simulink model "dtmf"  (Simulink 6.1)
settings: Solver=VariableStepDiscrete  StartTime=0  StopTime=5  RelTol=1e-3
PreLoadFcn:
  | Framesize=256,Fs=8192
values from neighbouring files (symbols this model uses):
  Fs = 8000    [generate.m]
undefined symbols (not defined in the file or in its folder): jet
libraries: dspddes3 x14, dspsrcs3 x5, dspsrcs2 x3, simulink3 x3, commutil2 x2, dspsigattribs x2, dspsigops x1, dsparch3 x1, dspswit3 x1, dspbuff3 x1, dspspect3 x1, dspsnks3 x1
settings Model: Creator=stuartm  LastModifiedBy=y  ExtModeTrigMode=oneshot  ExtModeArmWhenConnect=off  BufferReuse=off
settings DataIOCC: LimitDataPoints=off
settings OptimizationCC: BlockReduction=off  BooleanDataType=off  InlineInvariantSignals=off  OptimizeBlockIOStorage=off  BufferReuse=off  EnforceIntegerDowncast=off  ExpressionFolding=off  FoldNonRolledExpr=off  LocalBlockOutputs=off
settings HardwareCC: TargetUnknown=on

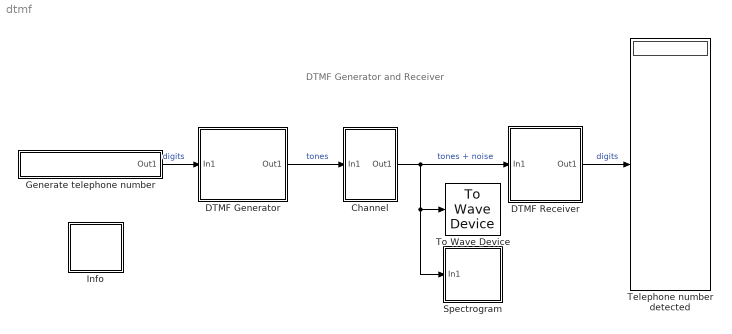
== system dtmf ==
  note: DTMF Generator and Receiver
  Channel : Subsystem  mask{var=.04, Fs=Fs, Framesize=Framesize, g=2}
      mask prompts: var "Noise power"; Fs "Sample Rate (Hz)"; g "Gain"
      mask Display: disp('Channel')
  DTMF Generator : Subsystem  mask{Fs=Fs, Framesize=Framesize}
      mask prompts: Fs "Sample Rate (Hz)"; Framesize "Framesize (Samples)"
      mask Display: disp('DTMF\nGenerator')
  DTMF Receiver : Subsystem  mask{Fs=Fs, Framesize=Framesize}
      mask prompts: Fs "Sample Rate"
      mask Display: disp('DTMF\nReceiver');
  Generate telephone number : Subsystem  mask{Number=[1 8 0 0 6 5 3 1 4 1 5], Td=(1/Fs)*256*6}
      mask prompts: Number "Telephone number"; Td "Digit Period (s)"
      mask Display: disp(Number)
  Info : Subsystem
      mask Display: disp('Info');
  Spectrogram : Subsystem
  Telephone number detected : Display
  To Wave Device : dspwin32/To Wave Device  bufDuration=1  initDelay=0.3  useDefaultDevice=on  userDeviceID=SoundMAX Digital Audio  enable24Bit=off
  wires:
  DTMF Generator/1(Out1) -> Channel/1(In1)  "tones"
  Generate telephone number/1(Out1) -> DTMF Generator/1(In1)  "digits"
  Channel/1(Out1) -> DTMF Receiver/1(In1), To Wave Device/1, Spectrogram/1(In1)  "tones + noise"
  DTMF Receiver/1(Out1) -> Telephone number detected/1  "digits"

== system dtmf/Channel ==
  In1 : Inport  Port=1  LatchInput=off
  Gain : Gain  Gain=g  SaturateOnIntegerOverflow=on
  Sum : Sum  Inputs=|++  SaturateOnIntegerOverflow=on  InputSameDT=on
  Vector of Noise : RandomNumber  Variance=var  Seed=[1:Framesize]  SampleTime=Framesize/Fs
  Out1 : Outport
  wires:
  In1/1 -> Gain/1
  Gain/1 -> Sum/1
  Vector of Noise/1 -> Sum/2
  Sum/1 -> Out1/1

== system dtmf/DTMF Generator ==
  In1 : Inport  Port=1  LatchInput=off
  Digit to Tone : Subsystem  TreatAsAtomicUnit=on
  Subtract  1 : Subsystem
  Out1 : Outport
  wires:
  Subtract  1/1(Out1) -> Digit to Tone/1(In1)
  In1/1 -> Subtract  1/1(In1), Digit to Tone/Enable
  Digit to Tone/1(Out1) -> Out1/1

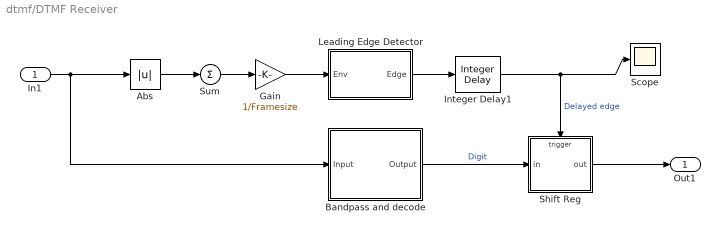
== system dtmf/DTMF Receiver ==
  In1 : Inport  Port=1  LatchInput=off
  Abs : Abs  SaturateOnIntegerOverflow=on
  Bandpass and decode : Subsystem
  Gain : Gain  Gain=1/Framesize  SaturateOnIntegerOverflow=on
  Integer Delay1 : dspsigops/Integer Delay  delay=1  ic=0
  Leading Edge Detector : Subsystem
  Scope : Scope
  Shift Reg : Stateflow chart  TreatAsAtomicUnit=on
  Sum : Sum  Inputs=1  SaturateOnIntegerOverflow=on  InputSameDT=on
  Out1 : Outport
  wires:
  In1/1 -> Bandpass and decode/1(Input), Abs/1
  Abs/1 -> Sum/1
  Sum/1 -> Gain/1
  Gain/1 -> Leading Edge Detector/1(Env)
  Shift Reg/1(out) -> Out1/1
  Integer Delay1/1 -> Shift Reg/Trigger, Scope/1  "Delayed edge"
  Bandpass and decode/1(Output) -> Shift Reg/1(in)  "Digit"
  Leading Edge Detector/1(Edge) -> Integer Delay1/1

== system dtmf/Generate telephone number ==
  Discrete Pulse Generator : DiscretePulseGenerator  SampleTime=Td
  Product : Product  SaturateOnIntegerOverflow=on  RndMeth=Zero  InputSameDT=on
  Triggered Signal From Workspace1 : dspsrcs3/Triggered Signal From Workspace  Signal=Number+1  TriggerType=Rising edge  ic=0  SamplesPerFrame=1  OutputAfterFinalValue=Setting To Zero
  Out1 : Outport
  wires:
  Discrete Pulse Generator/1 -> Product/1, Triggered Signal From Workspace1/Trigger
  Triggered Signal From Workspace1/1 -> Product/2
  Product/1 -> Out1/1

== system dtmf/Info ==
  note: DTMF Generator and Receiver
  note: This system uses the bandpass filter method of DTMF reception
      |
      | Enter a telephone number in first block
      |
      | "Telephone number detected" block shows last 12 digits detected

== system dtmf/Spectrogram ==
  In1 : Inport  Port=1  LatchInput=off
  Buffer2 : dspbuff3/Buffer  N=48  V=46  ic=-70
  Selector : Selector  Elements=1:Framesize/4  InputPortWidth=Framesize/2
  Short-Time FFT1 : dspspect3/Short-Time FFT  wintype=Hamming  Rs=50  beta=5  winsamp=Periodic  inheritFFT=off  fftsize=128  navg=2
  Spectogram : dspsnks3/Matrix Viewer  ImageParams=on  CMapStr=jet(256)  AxisColorbar=off  AxisParams=on  AxisOrigin=Lower left corner  XLabel=Time Index  YLabel=Frequency Index  ZLabel=dB Magnitude  FigPos=[54 474 312 203]  AxisZoom=off
      settings: YMin=-81.1042710009338  YMax=33.5779095386242
  To Workspace : ToWorkspace  VariableName=tones  SampleTime=-1  SaveFormat=Array
  Transpose : dspmtrx3/Transpose  Hermitian=off
  dB Conversion : dspmathops/dB Conversion  dBtype=dB  intype=Amplitude  R=1  fuzz=on
  wires:
  Short-Time FFT1/1 -> Selector/1
  Selector/1 -> dB Conversion/1
  Buffer2/1 -> Transpose/1
  dB Conversion/1 -> Buffer2/1
  In1/1 -> Short-Time FFT1/1, To Workspace/1
  Transpose/1 -> Spectogram/1

== system dtmf/DTMF Generator/Digit to Tone ==
  In1 : Inport  Port=1  LatchInput=off
  Enable : EnablePort
  Column Tones 1209Hz 1336Hz 1477Hz : Subsystem
  Column value for digit : Lookup  DialogController=Simulink.DDGSource  InputValues=[0 1 2 3 4 5 6 7 8 9 10 11]  OutputValues=[1 0 1 2 0 1 2 0 1 2 0 2]  SaturateOnIntegerOverflow=on
  "Row Tones 697Hz 770Hz 852Hz 941Hz " : Subsystem
  Row value for digit : Lookup  DialogController=Simulink.DDGSource  InputValues=[0 1 2 3 4 5 6 7 8 9 10 11]  OutputValues=[3 0 0 0 1 1 1 2 2 2 3 3]  SaturateOnIntegerOverflow=on
  Sum : Sum  Inputs=|+-  SaturateOnIntegerOverflow=on  InputSameDT=on
  Out1 : Outport  OutputWhenDisabled=reset  InitialOutput=0
  wires:
  Sum/1 -> Out1/1
  Column value for digit/1 -> Column Tones 1209Hz 1336Hz 1477Hz/1(Column)
  Row value for digit/1 -> "Row Tones 697Hz 770Hz 852Hz 941Hz "/1(Row)
  In1/1 -> Column value for digit/1, Row value for digit/1
  Column Tones 1209Hz 1336Hz 1477Hz/1(Tone) -> Sum/2
  "Row Tones 697Hz 770Hz 852Hz 941Hz "/1(Tone) -> Sum/1

== system dtmf/DTMF Generator/Subtract  1 ==
  In1 : Inport  Port=1  LatchInput=off
  Constant : Constant
  Sum : Sum  Inputs=|+-  SaturateOnIntegerOverflow=on  InputSameDT=on
  Out1 : Outport
  wires:
  Sum/1 -> Out1/1
  In1/1 -> Sum/1
  Constant/1 -> Sum/2

== system dtmf/DTMF Receiver/Bandpass and decode ==
  Input : Inport  Port=1  LatchInput=off
  Calculate Digit : simulink3/Functions & Tables/Look-Up Table (2-D)  x=[1:4]  y=[1:3]  t=[1 2 3;4 5 6;7 8 9;10 0 11]
  Calculate Column : Subsystem
  Calculate Row : Subsystem
  Output : Outport
  wires:
  Input/1 -> Calculate Column/1(In1), Calculate Row/1(In1)  "Input Tones"
  Calculate Digit/1 -> Output/1
  Calculate Row/1(Out1) -> Calculate Digit/1
  Calculate Column/1(Out1) -> Calculate Digit/2

== system dtmf/DTMF Receiver/Leading Edge Detector ==
  Env : Inport  Port=1  LatchInput=off
  Binary To Bipolar : Fcn  Expr=2*u-1
  Constant : Constant  Value=0.5
  Direct-Form II Transpose Filter : dsparch3/Direct-Form II Transpose Filter  num=[ones(1,4) -ones(1,4)]  den=1  ic=0
  Edge Detector1 : dspswit3/Edge Detector
  Relational Operator : RelationalOperator  InputSameDT=on
  Rising Edge Start : Fcn  Expr=u>5
  Edge : Outport  InitialOutput=0
  wires:
  Edge Detector1/1 -> Edge/1
  Direct-Form II Transpose Filter/1 -> Rising Edge Start/1
  Binary To Bipolar/1 -> Direct-Form II Transpose Filter/1
  Rising Edge Start/1 -> Edge Detector1/1
  Env/1 -> Relational Operator/1
  Constant/1 -> Relational Operator/2
  Relational Operator/1 -> Binary To Bipolar/1

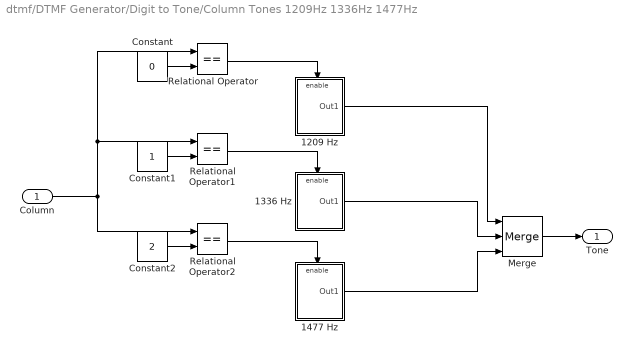
== system dtmf/DTMF Generator/Digit to Tone/Column Tones 1209Hz 1336Hz 1477Hz ==
  Column : Inport  Port=1  LatchInput=off
  1209 Hz : Subsystem  TreatAsAtomicUnit=on
  1336 Hz : Subsystem  TreatAsAtomicUnit=on
  1477 Hz : Subsystem  TreatAsAtomicUnit=on
  Constant : Constant  Value=0
  Constant1 : Constant
  Constant2 : Constant  Value=2
  Merge : Merge  Inputs=3
  Relational Operator : RelationalOperator  Operator===  InputSameDT=on
  Relational Operator1 : RelationalOperator  Operator===  InputSameDT=on
  Relational Operator2 : RelationalOperator  Operator===  InputSameDT=on
  Tone : Outport
  wires:
  Merge/1 -> Tone/1
  1477 Hz/1(Out1) -> Merge/3
  1336 Hz/1(Out1) -> Merge/2
  1209 Hz/1(Out1) -> Merge/1
  Column/1 -> Relational Operator/1, Relational Operator1/1, Relational Operator2/1
  Relational Operator/1 -> 1209 Hz/Enable
  Relational Operator1/1 -> 1336 Hz/Enable
  Relational Operator2/1 -> 1477 Hz/Enable
  Constant/1 -> Relational Operator/2
  Constant1/1 -> Relational Operator1/2
  Constant2/1 -> Relational Operator2/2

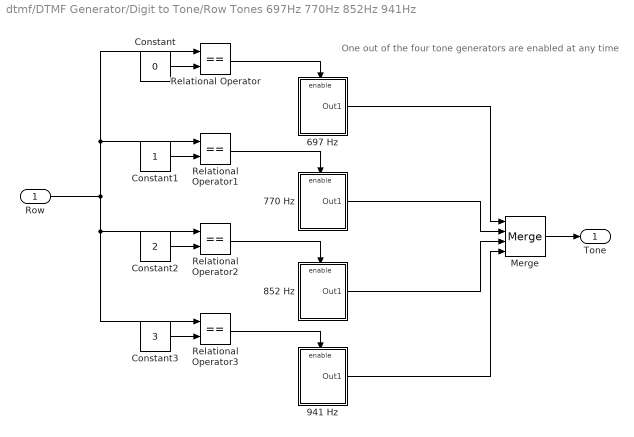
== system dtmf/DTMF Generator/Digit to Tone/Row Tones 697Hz 770Hz 852Hz 941Hz  ==
  note: One out of the four tone generators
      | are enabled at any time
  Row : Inport  Port=1  LatchInput=off
  697 Hz : Subsystem  TreatAsAtomicUnit=on
  770 Hz : Subsystem  TreatAsAtomicUnit=on
  852 Hz : Subsystem  TreatAsAtomicUnit=on
  941 Hz : Subsystem  TreatAsAtomicUnit=on
  Constant : Constant  Value=0
  Constant1 : Constant
  Constant2 : Constant  Value=2
  Constant3 : Constant  Value=3
  Merge : Merge  Inputs=4
  Relational Operator{,1..3} (4 alike) : RelationalOperator  Operator===  InputSameDT=on
  Tone : Outport
  wires:
  Row/1 -> Relational Operator/1, Relational Operator1/1, Relational Operator2/1, Relational Operator3/1
  697 Hz/1(Out1) -> Merge/1
  770 Hz/1(Out1) -> Merge/2
  852 Hz/1(Out1) -> Merge/3
  941 Hz/1(Out1) -> Merge/4
  Merge/1 -> Tone/1
  Relational Operator/1 -> 697 Hz/Enable
  Relational Operator1/1 -> 770 Hz/Enable
  Relational Operator2/1 -> 852 Hz/Enable
  Relational Operator3/1 -> 941 Hz/Enable
  Constant/1 -> Relational Operator/2
  Constant1/1 -> Relational Operator1/2
  Constant2/1 -> Relational Operator2/2
  Constant3/1 -> Relational Operator3/2

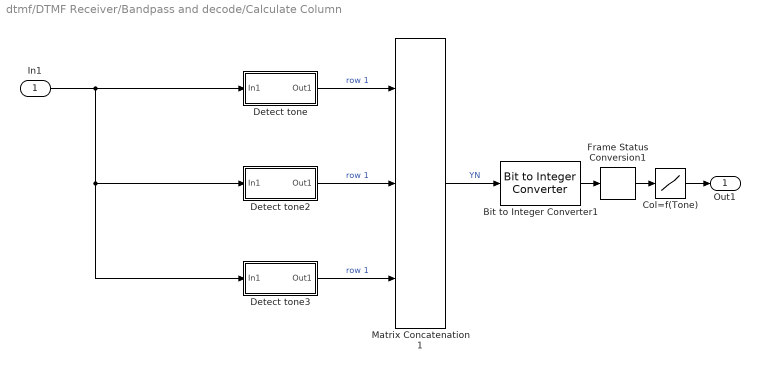
== system dtmf/DTMF Receiver/Bandpass and decode/Calculate Column ==
  In1 : Inport  Port=1  LatchInput=off
  Bit to Integer Converter1 : commutil2/Bit to Integer Converter  nbits=3
  Col=f(Tone) : Lookup  DialogController=Simulink.DDGSource  InputValues=[0:7]  OutputValues=[0 1 2 0 3 0 0 0]  SaturateOnIntegerOverflow=on
  Detect tone : Subsystem  mask{Fs=Fs, F=1477}
      mask prompts: Fs "Sample Rate (Hz)"; F "Frequency"
      settings: AttributesFormatString=%<F> Hz
  Detect tone2 : Subsystem  mask{Fs=Fs, F=1336}
      mask prompts: Fs "Sample Rate (Hz)"; F "Frequency"
      settings: AttributesFormatString=%<F> Hz
  Detect tone3 : Subsystem  mask{Fs=Fs, F=1209}
      mask prompts: Fs "Sample Rate (Hz)"; F "Frequency"
      settings: AttributesFormatString=%<F> Hz
  Frame Status Conversion1 : dspsigattribs/Frame Status Conversion  growRefPort=off  outframe=Sample-based
  Matrix Concatenation1 : simulink3/Signals & Systems/Matrix Concatenation  numInports=3  catMethod=Vertical
  Out1 : Outport
  wires:
  Matrix Concatenation1/1 -> Bit to Integer Converter1/1  "YN"
  Bit to Integer Converter1/1 -> Frame Status Conversion1/1
  Frame Status Conversion1/1 -> Col=f(Tone)/1
  Detect tone/1(Out1) -> Matrix Concatenation1/1  "row 1"
  Detect tone2/1(Out1) -> Matrix Concatenation1/2  "row 1"
  Detect tone3/1(Out1) -> Matrix Concatenation1/3  "row 1"
  In1/1 -> Detect tone2/1(In1), Detect tone3/1(In1), Detect tone/1(In1)
  Col=f(Tone)/1 -> Out1/1

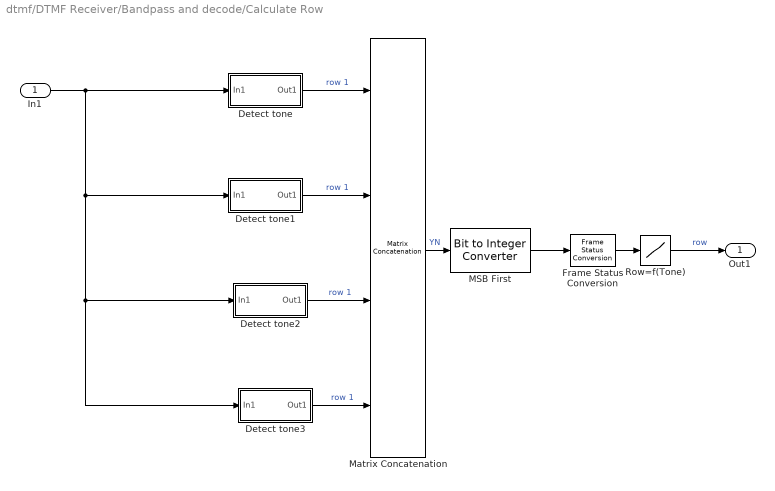
== system dtmf/DTMF Receiver/Bandpass and decode/Calculate Row ==
  In1 : Inport  Port=1  LatchInput=off
  Detect tone : Subsystem  mask{Fs=Fs, F=941}
      mask prompts: Fs "Sample Rate (Hz)"; F "Frequency"
      settings: AttributesFormatString=%<F> Hz
  Detect tone1 : Subsystem  mask{Fs=Fs, F=852}
      mask prompts: Fs "Sample Rate (Hz)"; F "Frequency"
      settings: AttributesFormatString=%<F> Hz
  Detect tone2 : Subsystem  mask{Fs=Fs, F=770}
      mask prompts: Fs "Sample Rate (Hz)"; F "Frequency"
      settings: AttributesFormatString=%<F> Hz
  Detect tone3 : Subsystem  mask{Fs=Fs, F=697}
      mask prompts: Fs "Sample Rate (Hz)"; F "Frequency"
      settings: AttributesFormatString=%<F> Hz
  Frame Status Conversion : dspsigattribs/Frame Status Conversion  growRefPort=off  outframe=Sample-based
  MSB First : commutil2/Bit to Integer Converter  nbits=4
  Matrix Concatenation : simulink3/Signals & Systems/Matrix Concatenation  numInports=4  catMethod=Vertical
  Row=f(Tone) : Lookup  DialogController=Simulink.DDGSource  InputValues=[0:15]  OutputValues=[0 1 2 0 3 0 0 0 4 0 0 0 0 0 0 0]  SaturateOnIntegerOverflow=on
  Out1 : Outport
  wires:
  Detect tone/1(Out1) -> Matrix Concatenation/1  "row 1"
  Matrix Concatenation/1 -> MSB First/1  "YN"
  MSB First/1 -> Frame Status Conversion/1
  Frame Status Conversion/1 -> Row=f(Tone)/1
  Detect tone1/1(Out1) -> Matrix Concatenation/2  "row 1"
  Detect tone2/1(Out1) -> Matrix Concatenation/3  "row 1"
  Detect tone3/1(Out1) -> Matrix Concatenation/4  "row 1"
  In1/1 -> Detect tone/1(In1), Detect tone1/1(In1), Detect tone2/1(In1), Detect tone3/1(In1)
  Row=f(Tone)/1 -> Out1/1  "row"

== system dtmf/DTMF Generator/Digit to Tone/Column Tones 1209Hz 1336Hz 1477Hz/1209 Hz ==
  Enable : EnablePort
  Sine Wave : dspsrcs2/Sine Wave  Amplitude=1  Frequency=1209  Phase=0  SampleMode=Discrete  OutComplex=Real  CompMethod=Trigonometric Fcn  SampleTime=1/Fs  SamplesPerFrame=Framesize  ResetState=Restart at time zero
  Out1 : Outport
  wires:
  Sine Wave/1 -> Out1/1

== system dtmf/DTMF Generator/Digit to Tone/Column Tones 1209Hz 1336Hz 1477Hz/1336 Hz ==
  Enable : EnablePort
  1336 Hz1 : dspsrcs2/Sine Wave  Amplitude=1  Frequency=1336  Phase=0  SampleMode=Discrete  OutComplex=Real  CompMethod=Trigonometric Fcn  SampleTime=1/Fs  SamplesPerFrame=Framesize  ResetState=Restart at time zero
  Out1 : Outport
  wires:
  1336 Hz1/1 -> Out1/1

== system dtmf/DTMF Generator/Digit to Tone/Column Tones 1209Hz 1336Hz 1477Hz/1477 Hz ==
  Enable : EnablePort
  1477 Hz1 : dspsrcs2/Sine Wave  Amplitude=1  Frequency=1477  Phase=0  SampleMode=Discrete  OutComplex=Real  CompMethod=Trigonometric Fcn  SampleTime=1/Fs  SamplesPerFrame=Framesize  ResetState=Restart at time zero
  Out1 : Outport
  wires:
  1477 Hz1/1 -> Out1/1

== system dtmf/DTMF Generator/Digit to Tone/Row Tones 697Hz 770Hz 852Hz 941Hz /697 Hz ==
  Enable : EnablePort
  Sine Wave : dspsrcs3/Sine Wave  Amplitude=1  Frequency=697  Phase=0  SampleMode=Discrete  OutComplex=Real  CompMethod=Trigonometric Fcn  TableSize=Speed  SampleTime=1/Fs  SamplesPerFrame=Framesize  ResetState=Restart at time zero
  Out1 : Outport
  wires:
  Sine Wave/1 -> Out1/1

== system dtmf/DTMF Generator/Digit to Tone/Row Tones 697Hz 770Hz 852Hz 941Hz /770 Hz ==
  Enable : EnablePort
  Sine Wave : dspsrcs3/Sine Wave  Amplitude=1  Frequency=770  Phase=0  SampleMode=Discrete  OutComplex=Real  CompMethod=Trigonometric Fcn  TableSize=Speed  SampleTime=1/Fs  SamplesPerFrame=Framesize  ResetState=Restart at time zero
  Out1 : Outport
  wires:
  Sine Wave/1 -> Out1/1

== system dtmf/DTMF Generator/Digit to Tone/Row Tones 697Hz 770Hz 852Hz 941Hz /852 Hz ==
  Enable : EnablePort
  Sine Wave : dspsrcs3/Sine Wave  Amplitude=1  Frequency=852  Phase=0  SampleMode=Discrete  OutComplex=Real  CompMethod=Trigonometric Fcn  TableSize=Speed  SampleTime=1/Fs  SamplesPerFrame=Framesize  ResetState=Restart at time zero
  Out1 : Outport
  wires:
  Sine Wave/1 -> Out1/1

== system dtmf/DTMF Generator/Digit to Tone/Row Tones 697Hz 770Hz 852Hz 941Hz /941 Hz ==
  Enable : EnablePort
  Sine Wave : dspsrcs3/Sine Wave  Amplitude=1  Frequency=941  Phase=0  SampleMode=Discrete  OutComplex=Real  CompMethod=Trigonometric Fcn  TableSize=Speed  SampleTime=1/Fs  SamplesPerFrame=Framesize  ResetState=Restart at time zero
  Out1 : Outport
  wires:
  Sine Wave/1 -> Out1/1

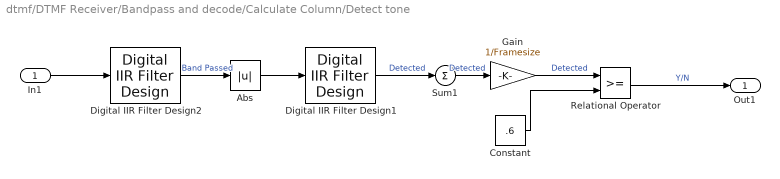
== system dtmf/DTMF Receiver/Bandpass and decode/Calculate Column/Detect tone ==
  In1 : Inport  Port=1  LatchInput=off
  Abs : Abs  SaturateOnIntegerOverflow=on
  Constant : Constant  Value=.6
  Digital IIR Filter Design1 : dspddes3/Digital IIR Filter Design  method=Butterworth  filttype=Lowpass  N=4  Wlo=100/(Fs/2)  Whi=(F+10)/(Fs/2)  Rp=1  Rs=20
  Digital IIR Filter Design2 : dspddes3/Digital IIR Filter Design  method=Chebyshev I  filttype=Bandpass  N=4  Wlo=(F-10)/(Fs/2)  Whi=(F+10)/(Fs/2)  Rp=1  Rs=20
  Gain : Gain  Gain=1/Framesize  SaturateOnIntegerOverflow=on
  Relational Operator : RelationalOperator  InputSameDT=on
  Sum1 : Sum  Inputs=1  SaturateOnIntegerOverflow=on  InputSameDT=on
  Out1 : Outport
  wires:
  Digital IIR Filter Design1/1 -> Sum1/1  "Detected"
  Relational Operator/1 -> Out1/1  "Y/N"
  Constant/1 -> Relational Operator/2
  Abs/1 -> Digital IIR Filter Design1/1
  Digital IIR Filter Design2/1 -> Abs/1  "Band Passed"
  In1/1 -> Digital IIR Filter Design2/1
  Sum1/1 -> Gain/1  "Detected"
  Gain/1 -> Relational Operator/1  "Detected"

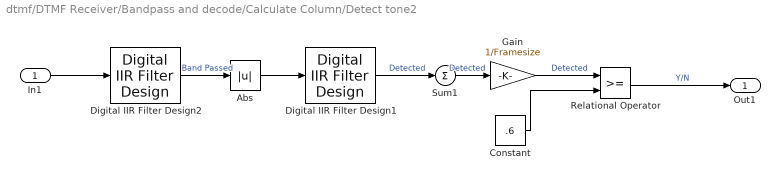
== system dtmf/DTMF Receiver/Bandpass and decode/Calculate Column/Detect tone2 ==
  In1 : Inport  Port=1  LatchInput=off
  Abs : Abs  SaturateOnIntegerOverflow=on
  Constant : Constant  Value=.6
  Digital IIR Filter Design1 : dspddes3/Digital IIR Filter Design  method=Butterworth  filttype=Lowpass  N=4  Wlo=100/(Fs/2)  Whi=(F+10)/(Fs/2)  Rp=1  Rs=20
  Digital IIR Filter Design2 : dspddes3/Digital IIR Filter Design  method=Chebyshev I  filttype=Bandpass  N=4  Wlo=(F-10)/(Fs/2)  Whi=(F+10)/(Fs/2)  Rp=1  Rs=20
  Gain : Gain  Gain=1/Framesize  SaturateOnIntegerOverflow=on
  Relational Operator : RelationalOperator  InputSameDT=on
  Sum1 : Sum  Inputs=1  SaturateOnIntegerOverflow=on  InputSameDT=on
  Out1 : Outport
  wires:
  Gain/1 -> Relational Operator/1  "Detected"
  Sum1/1 -> Gain/1  "Detected"
  In1/1 -> Digital IIR Filter Design2/1
  Digital IIR Filter Design2/1 -> Abs/1  "Band Passed"
  Abs/1 -> Digital IIR Filter Design1/1
  Constant/1 -> Relational Operator/2
  Relational Operator/1 -> Out1/1  "Y/N"
  Digital IIR Filter Design1/1 -> Sum1/1  "Detected"

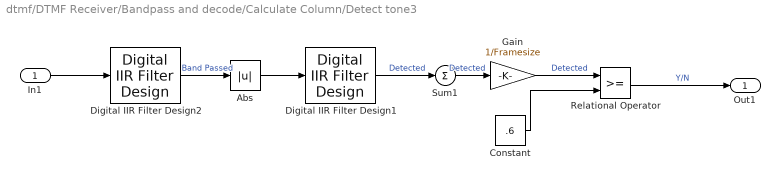
== system dtmf/DTMF Receiver/Bandpass and decode/Calculate Column/Detect tone3 ==
  In1 : Inport  Port=1  LatchInput=off
  Abs : Abs  SaturateOnIntegerOverflow=on
  Constant : Constant  Value=.6
  Digital IIR Filter Design1 : dspddes3/Digital IIR Filter Design  method=Butterworth  filttype=Lowpass  N=4  Wlo=100/(Fs/2)  Whi=(F+10)/(Fs/2)  Rp=1  Rs=20
  Digital IIR Filter Design2 : dspddes3/Digital IIR Filter Design  method=Chebyshev I  filttype=Bandpass  N=4  Wlo=(F-10)/(Fs/2)  Whi=(F+10)/(Fs/2)  Rp=1  Rs=20
  Gain : Gain  Gain=1/Framesize  SaturateOnIntegerOverflow=on
  Relational Operator : RelationalOperator  InputSameDT=on
  Sum1 : Sum  Inputs=1  SaturateOnIntegerOverflow=on  InputSameDT=on
  Out1 : Outport
  wires:
  Digital IIR Filter Design1/1 -> Sum1/1  "Detected"
  Relational Operator/1 -> Out1/1  "Y/N"
  Constant/1 -> Relational Operator/2
  Abs/1 -> Digital IIR Filter Design1/1
  Digital IIR Filter Design2/1 -> Abs/1  "Band Passed"
  In1/1 -> Digital IIR Filter Design2/1
  Sum1/1 -> Gain/1  "Detected"
  Gain/1 -> Relational Operator/1  "Detected"

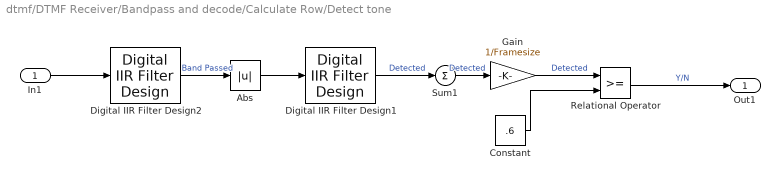
== system dtmf/DTMF Receiver/Bandpass and decode/Calculate Row/Detect tone ==
  In1 : Inport  Port=1  LatchInput=off
  Abs : Abs  SaturateOnIntegerOverflow=on
  Constant : Constant  Value=.6
  Digital IIR Filter Design1 : dspddes3/Digital IIR Filter Design  method=Butterworth  filttype=Lowpass  N=4  Wlo=100/(Fs/2)  Whi=(F+10)/(Fs/2)  Rp=1  Rs=20
  Digital IIR Filter Design2 : dspddes3/Digital IIR Filter Design  method=Chebyshev I  filttype=Bandpass  N=4  Wlo=(F-10)/(Fs/2)  Whi=(F+10)/(Fs/2)  Rp=1  Rs=20
  Gain : Gain  Gain=1/Framesize  SaturateOnIntegerOverflow=on
  Relational Operator : RelationalOperator  InputSameDT=on
  Sum1 : Sum  Inputs=1  SaturateOnIntegerOverflow=on  InputSameDT=on
  Out1 : Outport
  wires:
  Gain/1 -> Relational Operator/1  "Detected"
  Sum1/1 -> Gain/1  "Detected"
  In1/1 -> Digital IIR Filter Design2/1
  Digital IIR Filter Design2/1 -> Abs/1  "Band Passed"
  Abs/1 -> Digital IIR Filter Design1/1
  Constant/1 -> Relational Operator/2
  Relational Operator/1 -> Out1/1  "Y/N"
  Digital IIR Filter Design1/1 -> Sum1/1  "Detected"

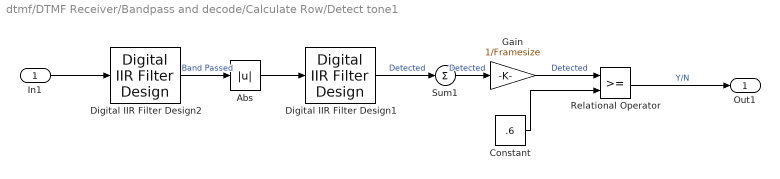
== system dtmf/DTMF Receiver/Bandpass and decode/Calculate Row/Detect tone1 ==
  In1 : Inport  Port=1  LatchInput=off
  Abs : Abs  SaturateOnIntegerOverflow=on
  Constant : Constant  Value=.6
  Digital IIR Filter Design1 : dspddes3/Digital IIR Filter Design  method=Butterworth  filttype=Lowpass  N=4  Wlo=100/(Fs/2)  Whi=(F+10)/(Fs/2)  Rp=1  Rs=20
  Digital IIR Filter Design2 : dspddes3/Digital IIR Filter Design  method=Chebyshev I  filttype=Bandpass  N=4  Wlo=(F-10)/(Fs/2)  Whi=(F+10)/(Fs/2)  Rp=1  Rs=20
  Gain : Gain  Gain=1/Framesize  SaturateOnIntegerOverflow=on
  Relational Operator : RelationalOperator  InputSameDT=on
  Sum1 : Sum  Inputs=1  SaturateOnIntegerOverflow=on  InputSameDT=on
  Out1 : Outport
  wires:
  Digital IIR Filter Design1/1 -> Sum1/1  "Detected"
  Relational Operator/1 -> Out1/1  "Y/N"
  Constant/1 -> Relational Operator/2
  Abs/1 -> Digital IIR Filter Design1/1
  Digital IIR Filter Design2/1 -> Abs/1  "Band Passed"
  In1/1 -> Digital IIR Filter Design2/1
  Sum1/1 -> Gain/1  "Detected"
  Gain/1 -> Relational Operator/1  "Detected"

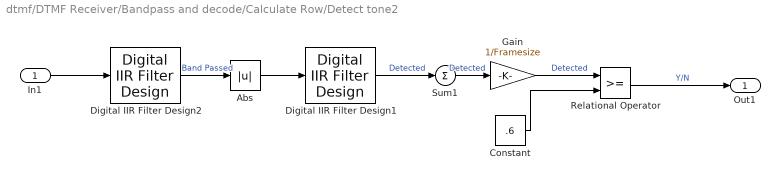
== system dtmf/DTMF Receiver/Bandpass and decode/Calculate Row/Detect tone2 ==
  In1 : Inport  Port=1  LatchInput=off
  Abs : Abs  SaturateOnIntegerOverflow=on
  Constant : Constant  Value=.6
  Digital IIR Filter Design1 : dspddes3/Digital IIR Filter Design  method=Butterworth  filttype=Lowpass  N=4  Wlo=100/(Fs/2)  Whi=(F+10)/(Fs/2)  Rp=1  Rs=20
  Digital IIR Filter Design2 : dspddes3/Digital IIR Filter Design  method=Chebyshev I  filttype=Bandpass  N=4  Wlo=(F-10)/(Fs/2)  Whi=(F+10)/(Fs/2)  Rp=1  Rs=20
  Gain : Gain  Gain=1/Framesize  SaturateOnIntegerOverflow=on
  Relational Operator : RelationalOperator  InputSameDT=on
  Sum1 : Sum  Inputs=1  SaturateOnIntegerOverflow=on  InputSameDT=on
  Out1 : Outport
  wires:
  Gain/1 -> Relational Operator/1  "Detected"
  Sum1/1 -> Gain/1  "Detected"
  In1/1 -> Digital IIR Filter Design2/1
  Digital IIR Filter Design2/1 -> Abs/1  "Band Passed"
  Abs/1 -> Digital IIR Filter Design1/1
  Constant/1 -> Relational Operator/2
  Relational Operator/1 -> Out1/1  "Y/N"
  Digital IIR Filter Design1/1 -> Sum1/1  "Detected"

== system dtmf/DTMF Receiver/Bandpass and decode/Calculate Row/Detect tone3 ==
  In1 : Inport  Port=1  LatchInput=off
  Abs : Abs  SaturateOnIntegerOverflow=on
  Constant : Constant  Value=.6
  Digital IIR Filter Design1 : dspddes3/Digital IIR Filter Design  method=Butterworth  filttype=Lowpass  N=4  Wlo=100/(Fs/2)  Whi=(F+10)/(Fs/2)  Rp=1  Rs=20
  Digital IIR Filter Design2 : dspddes3/Digital IIR Filter Design  method=Chebyshev I  filttype=Bandpass  N=4  Wlo=(F-10)/(Fs/2)  Whi=(F+10)/(Fs/2)  Rp=1  Rs=20
  Gain : Gain  Gain=1/Framesize  SaturateOnIntegerOverflow=on
  Relational Operator : RelationalOperator  InputSameDT=on
  Sum1 : Sum  Inputs=1  SaturateOnIntegerOverflow=on  InputSameDT=on
  Out1 : Outport
  wires:
  Digital IIR Filter Design1/1 -> Sum1/1  "Detected"
  Relational Operator/1 -> Out1/1  "Y/N"
  Constant/1 -> Relational Operator/2
  Abs/1 -> Digital IIR Filter Design1/1
  Digital IIR Filter Design2/1 -> Abs/1  "Band Passed"
  In1/1 -> Digital IIR Filter Design2/1
  Sum1/1 -> Gain/1  "Detected"
  Gain/1 -> Relational Operator/1  "Detected"

== stateflow chart DTMF Receiver/Shift Reg ==
  settings: executeAtInitialization=1
  state On
    On -> (junction 4) : CLK{i=0;}
    (junction 4) -> (junction 5) : {out[i]=out[i+1];}
    (junction 5) -> (junction 6) : {out[10]=in;}
    (junction 5) -> (junction 4) : [i<9]{i++;}
  (default) -> On
  data: i local double; in input double; out output double size=11
  events: CLK input RISING_EDGE_EVENT
